simulink model "Ex3Simulink"  (R2017a)
settings: Solver=VariableStepAuto  StartTime=0.0  StopTime=10.0  RelTol=1e-3
values from neighbouring files (symbols this model uses):
  dm = 3.8e-6    (= 3.8e-06)    [ex3Parameters.m]
  J = (n*n*Jr + Jl) / n    (= 3.7300072)    [ex3Parameters.m]
  Ke = Kt / 9.55    (= 0.00729842931937)    [ex3Parameters.m]
  Kt = 69.7e-3    (= 0.0697)    [ex3Parameters.m]
  n = 5    [ex3Parameters.m]
  R = 112    [ex3Parameters.m]
settings Model: Creator=99641  LastModifiedBy=99641

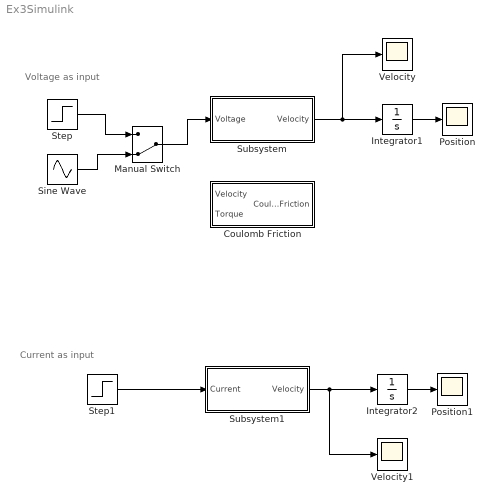
== system Ex3Simulink ==
  note: Current as input
  note: Voltage as input
  Coulomb Friction : Subsystem
  Integrator1 : Integrator
  Integrator2 : Integrator
  Manual Switch : ManualSwitch  CurrentSetting=0
  Position : Scope
  Position1 : Scope
  Sine Wave : Sin  Amplitude=10  SampleTime=0
  Step : Step  After=10  SampleTime=0
  Step1 : Step  SampleTime=0
  Subsystem : Subsystem
  Subsystem1 : Subsystem
  Velocity : Scope
  Velocity1 : Scope
  wires:
  Subsystem1/1("Velocity ") -> Integrator2/1, Velocity1/1
  Step1/1 -> Subsystem1/1(Current)
  Subsystem/1("Velocity ") -> Velocity/1, Integrator1/1
  Integrator2/1 -> Position1/1
  Integrator1/1 -> Position/1
  Step/1 -> Manual Switch/1
  Sine Wave/1 -> Manual Switch/2
  Manual Switch/1 -> Subsystem/1(Voltage)

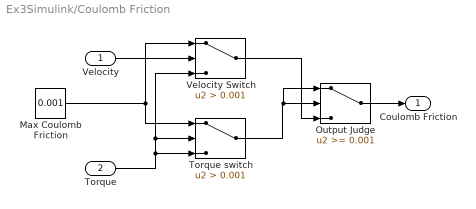
== system Ex3Simulink/Coulomb Friction ==
  Velocity : Inport
  Torque : Inport  Port=2
  Max Coulomb Friction : Constant  Value=0.001
  Output Judge : Switch  Threshold=0.001
  Torque switch : Switch  Criteria=u2 > Threshold  Threshold=0.001
  "Velocity Switch " : Switch  Criteria=u2 > Threshold  Threshold=0.001
  Coulomb Friction : Outport
  wires:
  Velocity/1 -> "Velocity Switch "/2
  Torque switch/1 -> Output Judge/1, Output Judge/2
  Output Judge/1 -> Coulomb Friction/1
  Torque/1 -> Torque switch/3, "Velocity Switch "/3, Torque switch/2
  Max Coulomb Friction/1 -> Torque switch/1, "Velocity Switch "/1
  "Velocity Switch "/1 -> Output Judge/3

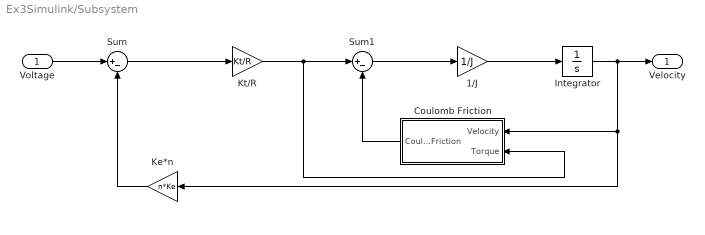
== system Ex3Simulink/Subsystem ==
  Voltage : Inport
  1/J : Gain  Gain=1/J
  Coulomb Friction : Subsystem
  Integrator : Integrator
  Ke*n : Gain  Gain=n*Ke
  Kt/R : Gain  Gain=Kt/R
  Sum : Sum  Inputs=|+-
  Sum1 : Sum  Inputs=|+-
  "Velocity " : Outport
  wires:
  Voltage/1 -> Sum/1
  Sum/1 -> Kt/R/1
  Sum1/1 -> 1/J/1
  Kt/R/1 -> Coulomb Friction/2(Torque), Sum1/1
  1/J/1 -> Integrator/1
  Integrator/1 -> Ke*n/1, Coulomb Friction/1(Velocity), "Velocity "/1
  Ke*n/1 -> Sum/2
  Coulomb Friction/1(Coulomb Friction) -> Sum1/2

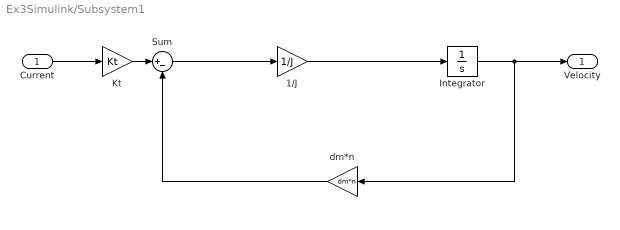
== system Ex3Simulink/Subsystem1 ==
  Current : Inport
  1/J : Gain  Gain=1/J
  Integrator : Integrator
  Kt : Gain  Gain=Kt
  Sum : Sum  Inputs=|+-
  dm*n : Gain  Gain=dm*n
  "Velocity " : Outport
  wires:
  dm*n/1 -> Sum/2
  Integrator/1 -> "Velocity "/1, dm*n/1
  1/J/1 -> Integrator/1
  Sum/1 -> 1/J/1
  Current/1 -> Kt/1
  Kt/1 -> Sum/1

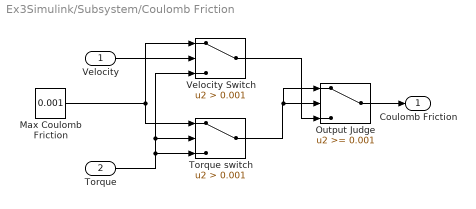
== system Ex3Simulink/Subsystem/Coulomb Friction ==
  Velocity : Inport
  Torque : Inport  Port=2
  Max Coulomb Friction : Constant  Value=0.001
  Output Judge : Switch  Threshold=0.001
  Torque switch : Switch  Criteria=u2 > Threshold  Threshold=0.001
  "Velocity Switch " : Switch  Criteria=u2 > Threshold  Threshold=0.001
  Coulomb Friction : Outport
  wires:
  Velocity/1 -> "Velocity Switch "/2
  Torque switch/1 -> Output Judge/1, Output Judge/2
  Output Judge/1 -> Coulomb Friction/1
  Torque/1 -> Torque switch/3, "Velocity Switch "/3, Torque switch/2
  Max Coulomb Friction/1 -> Torque switch/1, "Velocity Switch "/1
  "Velocity Switch "/1 -> Output Judge/3
